simulink model "VU_lineFollow1b"  (Simulink 10.0)
settings: Solver=FixedStepDiscrete  StartTime=0.0  StopTime=inf  FixedStep=0.05  RelTol=1e-3  EnableMultiTasking=on
libraries: lego_nxt_lib x6
settings Model: Creator=jpeytonj  LastModifiedBy=bhisma
settings DataIOCC: LimitDataPoints=on  SignalLoggingSaveFormat=ModelDataLogs
settings OptimizationCC: ExpressionDepthLimit=2147483647
settings DebuggingCC: SolverPrmCheckMsg=warning  FcnCallInpInsideContextMsg=warning  StateNameClashWarn=warning
settings SFSimCC: SimParseCustomCode=off
settings RTWCC: Description=Lego NXT Real-Time Target  SystemTargetFile=lrt.tlc  GenCodeOnly=on  TemplateMakefile=lrt_ecrobot.tmf
settings STFCustomTargetCC: ModelReferenceCompliant=off  GeneratePreprocessorConditionals=Disable all  MatFileLogging=on  CPPClassGenCompliant=on  SystemTargetFile=lrt.tlc
settings GRTTargetCC: ModelReferenceCompliant=off  ParMdlRefBuildCompliant=off  CompOptLevelCompliant=off  ConcurrentExecutionCompliant=off  GeneratePreprocessorConditionals=Disable all  UseToolchainInfoCompliant=off  ExtModeMexFile=ext_serial_win32_comm
settings CustomProperty: DataType=RTWOptions_EnumType_C__RTtools_VU-LRT_lrt_1codeGenType  Value=Integer-only
settings EnumStrPairs: String=Integer-only
settings ConfigComp: CovExternalEMLEnable=off

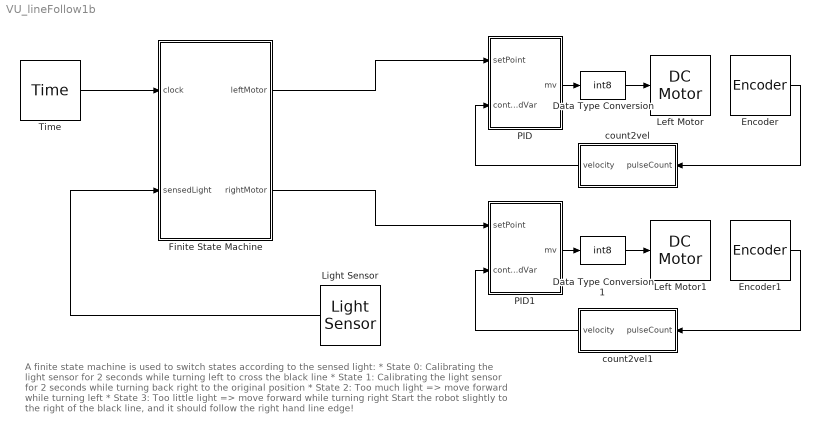
== system VU_lineFollow1b ==
  note: A finite state machine is used to switch states according to the sensed light:
      | * State 0:  Calibrating the light sensor for 2 seconds while turning left to cross the black line
      | * State 1:  Calibrating the light sensor for 2 seconds while turning back right to the original position
      | * State 2:  Too much light => move forward while turning left
      | * State 3:  Too little light => move forward while turning right
      | Start the robot slightly to the right of the black line, and it should follow the right hand line edge!
  Data Type Conversion : DataTypeConversion  OutDataTypeStr=int8  SaturateOnIntegerOverflow=on
  Data Type Conversion1 : DataTypeConversion  OutDataTypeStr=int8  SaturateOnIntegerOverflow=on
  Encoder : lego_nxt_lib/Encoder  port=Port C  st=0.05
  Encoder1 : lego_nxt_lib/Encoder  port=Port B  st=0.05
  Finite State Machine : MATLAB Function  TreatAsAtomicUnit=on
  Left Motor : lego_nxt_lib/DC Motor  port=Port C  brake=Coast
  Left Motor1 : lego_nxt_lib/DC Motor  port=Port B  brake=Coast
  Light Sensor : lego_nxt_lib/Light Sensor  port=Port 3  st=0.05
  PID : Subsystem  mask{Kc=10, Ti=0.4, Td=0, mvMax=100, mvMin=-100}
      mask prompts: Kc "Proportional gain:"; Ti "Integral time:"; Td "Derivative time:"; mvMax "Max manipulated output Limit:"; mvMin "Min manipulated output Limit:"
  PID1 : Subsystem  mask{Kc=10, Ti=0.4, Td=0, mvMax=100, mvMin=-100}
      mask prompts: Kc "Proportional gain:"; Ti "Integral time:"; Td "Derivative time:"; mvMax "Max manipulated output Limit:"; mvMin "Min manipulated output Limit:"
  Time : lego_nxt_lib/Time  st=0.05
  count2vel : Subsystem  mask(count2vel){gainFactor=1/0.05*1/360}
      mask prompts: gainFactor "Gain Factor:"
      mask help:
      | Use gainFactor to define units of the result:
      | If gainFactor=1, => units of velocity= (pulses/sample).
      | The encoders give 360 pulses / revolution of the output shaft
      |
      | Example:  To obtain velocity in rev/sec
      | velocity = (pulses/sample) * (samples/sec) * (rev/pulses) = rev/sec
      | Given a sample period T=0.1, and the known 360 pulses per rev...
      | => gainFactor = (1/0.1) * (1/360) = 1/36
      |
      | Not clear what happens when the pulse count overflows
  count2vel1 : Subsystem  mask(count2vel){gainFactor=1/0.05*1/360}
      mask prompts: gainFactor "Gain Factor:"
      mask help:
      | Use gainFactor to define units of the result:
      | If gainFactor=1, => units of velocity= (pulses/sample).
      | The encoders give 360 pulses / revolution of the output shaft
      |
      | Example:  To obtain velocity in rev/sec
      | velocity = (pulses/sample) * (samples/sec) * (rev/pulses) = rev/sec
      | Given a sample period T=0.1, and the known 360 pulses per rev...
      | => gainFactor = (1/0.1) * (1/360) = 1/36
      |
      | Not clear what happens when the pulse count overflows
  wires:
  Light Sensor/1 -> Finite State Machine/2(sensedLight)
  Time/1 -> Finite State Machine/1(clock)
  PID/1(mv) -> Data Type Conversion/1
  Data Type Conversion/1 -> Left Motor/1
  Encoder/1 -> count2vel/1(pulseCount)
  count2vel/1(velocity) -> PID/2(controlledVar)
  PID1/1(mv) -> Data Type Conversion1/1
  Data Type Conversion1/1 -> Left Motor1/1
  Encoder1/1 -> count2vel1/1(pulseCount)
  count2vel1/1(velocity) -> PID1/2(controlledVar)
  Finite State Machine/1(leftMotor) -> PID/1(setPoint)
  Finite State Machine/2(rightMotor) -> PID1/1(setPoint)

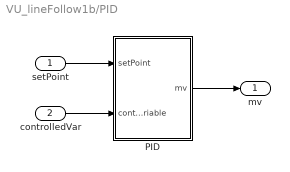
== system VU_lineFollow1b/PID ==
  setPoint : Inport
  controlledVar : Inport  Port=2
  PID : MATLAB Function  TreatAsAtomicUnit=on
  mv : Outport
  wires:
  PID/1(mv) -> mv/1
  controlledVar/1 -> PID/2(contolledVariable)
  setPoint/1 -> PID/1(setPoint)

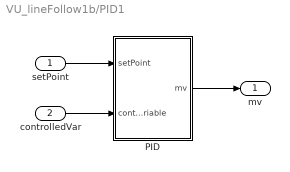
== system VU_lineFollow1b/PID1 ==
  setPoint : Inport
  controlledVar : Inport  Port=2
  PID : MATLAB Function  TreatAsAtomicUnit=on
  mv : Outport
  wires:
  PID/1(mv) -> mv/1
  controlledVar/1 -> PID/2(contolledVariable)
  setPoint/1 -> PID/1(setPoint)

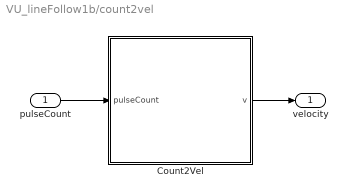
== system VU_lineFollow1b/count2vel ==
  pulseCount : Inport
  Count2Vel : MATLAB Function  TreatAsAtomicUnit=on
  velocity : Outport
  wires:
  Count2Vel/1(v) -> velocity/1
  pulseCount/1 -> Count2Vel/1(pulseCount)

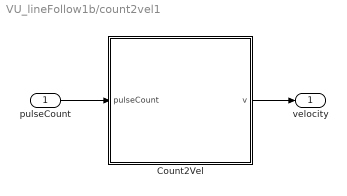
== system VU_lineFollow1b/count2vel1 ==
  pulseCount : Inport
  Count2Vel : MATLAB Function  TreatAsAtomicUnit=on
  velocity : Outport
  wires:
  Count2Vel/1(v) -> velocity/1
  pulseCount/1 -> Count2Vel/1(pulseCount)

== matlab function PID/PID ==
  data: setPoint input double; mv output double; contolledVariable input double; Kc parameter double; Ti parameter double; Td parameter double; mvMax parameter double; mvMin parameter double
function mv= PID (setPoint,contolledVariable,Kc,Ti,Td,mvMax,mvMin)

% PID uses the 'velocity algorithm' to drive the 
% 'controlledVariable' to follow the 'setPoint'  
% The manipulated variable is limited between 'mvMax' and 'mvMin'
% The controller proportional, integral and derivative gains are Kc, Ti, Td

% Date: 1 Oct 2010
% Author: JC Peyton Jones
% Villanova University

% Initialize persistent variables
persistent ekm1 ekm2 mvm1

if (isempty(ekm1)),
    ekm1= 0;        % e(k-1) is the error at time k-1
    ekm2= 0;        % e(k-2) is the error at time k-2
    mvm1= 0;        % mv(k-1) is the manipulated variable at k-1
end

% Compute the control action (the manipulated variable)
ek= setPoint - contolledVariable;
dm = Kc*(ek-ekm1 + (1/Ti)*ek + Td*(ek - 2*ekm1 + ekm2));
mv = mvm1 + dm;

% Limit the control action
if (mv > mvMax),
    mv = mvMax;
elseif (mv < mvMin),
    mv = mvMin;
end;

% Shift variables ready for next time
ekm2= ekm1;     % e(k-2)= e(k-1);
ekm1= ek;       % e(k-1)= e(k);
mvm1= mv;       % mv(k-1)= mv;

== matlab function Finite State Machine ==
  data: clock input double; sensedLight input double; leftMotor output double; rightMotor output double
function [leftMotor, rightMotor] = fsm(clock, sensedLight)

persistent currentState maxLight minLight threshold 

if isempty(currentState),
    currentState= uint8(0);
    maxLight= uint16(0);
    minLight= uint16(1023);
    threshold= uint16(45);
end;

leftMotor= 0;
rightMotor= 0;

switch currentState
    case 0 %Calibration - turning left
        leftMotor= -0.4;
        rightMotor= 0.4;
        if sensedLight>maxLight, maxLight= sensedLight; end;
        if sensedLight<minLight, minLight= sensedLight; end;
        if (clock>500), currentState= uint8(1); end;
    case 1 %Calibration - turning right
        leftMotor= 0.4;
        rightMotor= -0.4;
        if sensedLight>maxLight, maxLight= sensedLight; end;
        if sensedLight<minLight, minLight= sensedLight; end;
        if (clock>1400), 
            threshold = (maxLight + minLight)/2;
            currentState= uint8(2); 
        end;
    case 2 %Too much light => turn Left
        leftMotor= 0.4;
        rightMotor= 1.0;
        if sensedLight<threshold, currentState= uint8(3); end;
    case 3 %Too little light => turn Right
        leftMotor= 1.0;
        rightMotor= 0.4;
        if sensedLight>threshold, currentState= uint8(2); end;
end

== matlab function PID1/PID ==
  data: setPoint input double; mv output double; contolledVariable input double; Kc parameter double; Ti parameter double; Td parameter double; mvMax parameter double; mvMin parameter double
function mv= PID (setPoint,contolledVariable,Kc,Ti,Td,mvMax,mvMin)

% PID uses the 'velocity algorithm' to drive the 
% 'controlledVariable' to follow the 'setPoint'  
% The manipulated variable is limited between 'mvMax' and 'mvMin'
% The controller proportional, integral and derivative gains are Kc, Ti, Td

% Date: 1 Oct 2010
% Author: JC Peyton Jones
% Villanova University

% Initialize persistent variables
persistent ekm1 ekm2 mvm1

if (isempty(ekm1)),
    ekm1= 0;        % e(k-1) is the error at time k-1
    ekm2= 0;        % e(k-2) is the error at time k-2
    mvm1= 0;        % mv(k-1) is the manipulated variable at k-1
end

% Compute the control action (the manipulated variable)
ek= setPoint - contolledVariable;
dm = Kc*(ek-ekm1 + (1/Ti)*ek + Td*(ek - 2*ekm1 + ekm2));
mv = mvm1 + dm;

% Limit the control action
if (mv > mvMax),
    mv = mvMax;
elseif (mv < mvMin),
    mv = mvMin;
end;

% Shift variables ready for next time
ekm2= ekm1;     % e(k-2)= e(k-1);
ekm1= ek;       % e(k-1)= e(k);
mvm1= mv;       % mv(k-1)= mv;

== matlab function count2vel1/Count2Vel ==
  data: pulseCount input double; v output double; gainFactor parameter double
function v= velocity (pulseCount,gainFactor)

% Velocity computes the velocity in engineering units defined by gainFactor
% If gainFactor=1, => units are pulses/sample.  There are 360 pulses per rev
%
% Example:  To obtain velocity in rev/sec
% velocity = (pulses/sample) * (samples/sec) * (rev/pulses) = rev/sec
% Given a sample period T=0.1, and the known 360 pulses per rev...
% => gainFactor = (1/0.1) * (1/360) = 1/36
%
% Not clear what happens when the pulse count overflows


% Initialize persistent variables
persistent prevPulseCount

if (isempty(prevPulseCount)),
    prevPulseCount= int32(0); 
end

% Compute the velocity in units defined by gainFactor
v= double(pulseCount - prevPulseCount) * gainFactor;
prevPulseCount= pulseCount;

== matlab function count2vel/Count2Vel ==
  data: pulseCount input double; v output double; gainFactor parameter double
function v= velocity (pulseCount,gainFactor)

% Velocity computes the velocity in engineering units defined by gainFactor
% If gainFactor=1, => units are pulses/sample.  There are 360 pulses per rev
%
% Example:  To obtain velocity in rev/sec
% velocity = (pulses/sample) * (samples/sec) * (rev/pulses) = rev/sec
% Given a sample period T=0.1, and the known 360 pulses per rev...
% => gainFactor = (1/0.1) * (1/360) = 1/36
%
% Not clear what happens when the pulse count overflows


% Initialize persistent variables
persistent prevPulseCount

if (isempty(prevPulseCount)),
    prevPulseCount= int32(0); 
end

% Compute the velocity in units defined by gainFactor
v= double(pulseCount - prevPulseCount) * gainFactor;
prevPulseCount= pulseCount;
